simulink model "dcmtrCtrl_PID_wHandCode"  (R2022a)
settings: configuration reference "mtrCtrl_config" (kept outside this file)
settings Model: DataDictionary=dcmtr_ctrl.sldd  Creator=smuckati  LastModifiedBy=smuckati
settings ConfigSetRef: SourceName=mtrCtrl_config

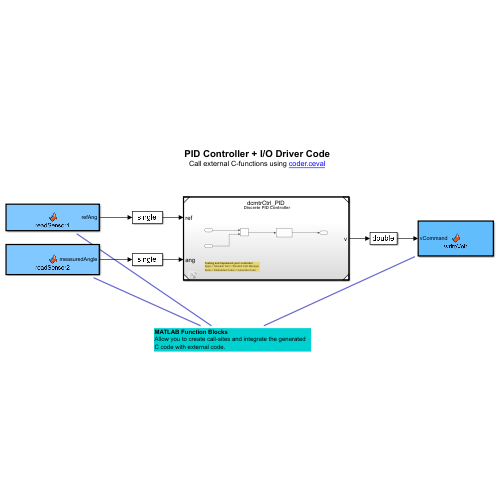
[thumbnail: Simulink's stored preview of the top-level diagram]
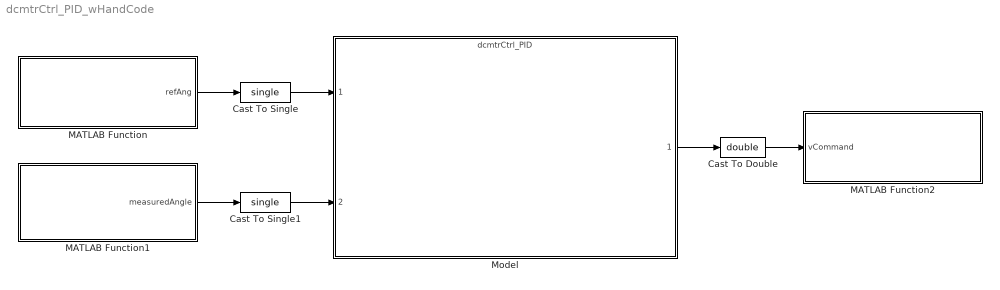
== system dcmtrCtrl_PID_wHandCode ==
  Cast To Double : DataTypeConversion  OutDataTypeStr=double  SaturateOnIntegerOverflow=off  RndMeth=Floor
  Cast To Single : DataTypeConversion  OutDataTypeStr=single  SaturateOnIntegerOverflow=off  RndMeth=Floor
  Cast To Single1 : DataTypeConversion  OutDataTypeStr=single  SaturateOnIntegerOverflow=off  RndMeth=Floor
  MATLAB Function : MATLAB Function  TreatAsAtomicUnit=on
  MATLAB Function1 : MATLAB Function  TreatAsAtomicUnit=on
  MATLAB Function2 : MATLAB Function  TreatAsAtomicUnit=on
  Model : ModelReference  ModelNameDialog=dcmtrCtrl_PID.slx  SimulationMode=Normal  ModelReferenceVersion=2.1
  wires:
  MATLAB Function/1(refAng) -> Cast To Single/1
  Cast To Single/1 -> Model/1
  Cast To Single1/1 -> Model/2
  MATLAB Function1/1(measuredAngle) -> Cast To Single1/1
  Model/1 -> Cast To Double/1
  Cast To Double/1 -> MATLAB Function2/1(vCommand)

== matlab function dcmtrCtrl_PID_wHandCode/MATLAB Function1 ==
  data: measuredAngle output
function measuredAngle = readSensor2

    coder.extrinsic('handCodeDir');
    % Function called "handCodeDir" is located in the same directlory as
    % the C files. coder.extrinsic ensures you can call this function to
    % return the directory location info back.
    
    measuredAngle  = 0;
    
    if( coder.target( 'Rtw' ) )
        customDir = coder.const(handCodeDir); % location of C files

        coder.cinclude( 'hand_code_header.h' );
        coder.updateBuildInfo( 'addIncludePaths', customDir );
        coder.updateBuildInfo( 'addSourceFiles', 'hand_code_source.c' );
        coder.updateBuildInfo( 'addSourcePaths', customDir );
        
        measuredAngle = coder.ceval( 'get_measuredAngle' );
        
    else
        % Use the initial values for simulation.
    end
    
    return;
end

== matlab function dcmtrCtrl_PID_wHandCode/MATLAB Function ==
  data: refAng output
function refAng = readSensor1

    coder.extrinsic('handCodeDir');
    % Function called "handCodeDir" is located in the same directlory as
    % the C files. coder.extrinsic ensures you can call this function to
    % return the directory location info back.
    
    refAng = pi/3;
    
    if( coder.target( 'Rtw' ) )
        customDir = coder.const(handCodeDir); % location of C files
        
        coder.cinclude( 'hand_code_header.h' );
        coder.updateBuildInfo( 'addIncludePaths', customDir );
        coder.updateBuildInfo( 'addSourceFiles', 'hand_code_source.c' );
        coder.updateBuildInfo( 'addSourcePaths', customDir );
        
        refAng = coder.ceval( 'get_motor_refAngle' );
        
    else
        % Use the initial values for simulation.
    end
    
    return;
end

== matlab function dcmtrCtrl_PID_wHandCode/MATLAB Function2 ==
  data: vCommand input
function writeVolt(vCommand)

    coder.extrinsic('handCodeDir');
    % Function called "handCodeDir" is located in the same directlory as
    % the C files. coder.extrinsic ensures you can call this function to
    % return the directory location info back.
    
    if( coder.target( 'Rtw' ) )
        customDir = coder.const(handCodeDir); % location of C files
        
        coder.cinclude( 'hand_code_header.h' );
        coder.updateBuildInfo( 'addIncludePaths', customDir );
        coder.updateBuildInfo( 'addSourceFiles', 'hand_code_source.c' );
        coder.updateBuildInfo( 'addSourcePaths', customDir );
        
        coder.ceval( 'request_mtrCmd' , vCommand );
        
    else
        % Use the initial values for simulation.
    end
    
    return;
end
